simulink model "bisezione"  (R2017a)
settings: Solver=FixedStepDiscrete  StartTime=0.0  StopTime=inf  FixedStep=1  RelTol=1e-3
values from neighbouring files (symbols this model uses):
  a = -3    [bisezioneSimulink.m]
  b = 5    [bisezioneSimulink.m]
  tol = 1e-3    (= 0.001)    [bisezioneSimulink.m]    (also in zero_funzione.m)
libraries: simulink x1
settings Model: Creator=Enrico Donato  LastModifiedBy=Enrico Donato

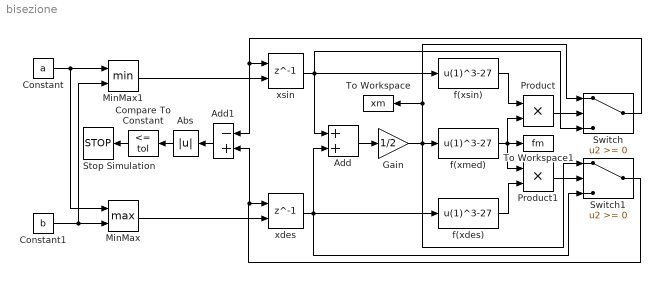
== system bisezione ==
  Abs : Abs
  Add : Sum
  Add1 : Sum  Inputs=-+
  Compare To Constant : simulink/Logic and Bit Operations/Compare To Constant  relop=<=  const=tol  OutDataTypeStr=boolean
  Constant : Constant  Value=a
  Constant1 : Constant  Value=b
  Gain : Gain  Gain=1/2
  MinMax : MinMax  Function=max  Inputs=2
  MinMax1 : MinMax  Inputs=2
  Product : Product
  Product1 : Product
  Stop Simulation : Stop
  Switch : Switch
  Switch1 : Switch
  To Workspace : ToWorkspace  VariableName=xm  SampleTime=-1
      settings: Save2DSignal=2-D array (concatenate along first dimension)
  To Workspace1 : ToWorkspace  VariableName=fm  SampleTime=-1
      settings: Save2DSignal=2-D array (concatenate along first dimension)
  f(xdes) : Fcn  Expr=u(1)^3-27
  f(xmed) : Fcn  Expr=u(1)^3-27
  f(xsin) : Fcn  Expr=u(1)^3-27
  xdes : Delay  DelayLength=1  InitialConditionSource=Input port  InitialCondition=0
      settings: InputPortMap=u0,p4
  xsin : Delay  DelayLength=1  InitialConditionSource=Input port  InitialCondition=0
      settings: InputPortMap=u0,p4
  wires:
  Constant/1 -> MinMax/1, MinMax1/1
  Constant1/1 -> MinMax/2, MinMax1/2
  MinMax/1 -> xdes/2
  MinMax1/1 -> xsin/2
  xdes/1 -> Switch1/3, f(xdes)/1, Add/2
  Add/1 -> Gain/1
  Gain/1 -> f(xmed)/1, Switch/1, To Workspace/1, Switch1/1
  f(xmed)/1 -> To Workspace1/1, Product1/1, Product/2
  f(xsin)/1 -> Product/1
  f(xdes)/1 -> Product1/2
  xsin/1 -> Switch/3, f(xsin)/1, Add/1
  Switch/1 -> xsin/1, Add1/1
  Switch1/1 -> Add1/2, xdes/1
  Product/1 -> Switch/2
  Product1/1 -> Switch1/2
  Add1/1 -> Abs/1
  Abs/1 -> Compare To Constant/1
  Compare To Constant/1 -> Stop Simulation/1
